simulink model "low_pass_filter"  (R2024b)
settings: Solver=FixedStepAuto  StartTime=0.0  StopTime=20  FixedStep=0.01  RelTol=1e-3
values from neighbouring files (symbols this model uses):
  alpha = 0.1    [lowpass_constants.m]
settings Model: Creator=AKhmad  LastModifiedBy=AKhmad

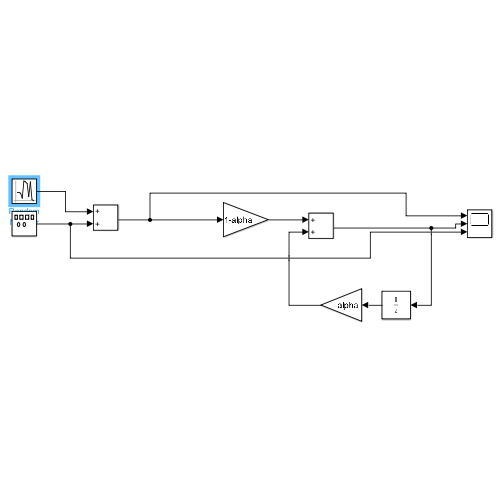
[thumbnail: Simulink's stored preview of the top-level diagram]
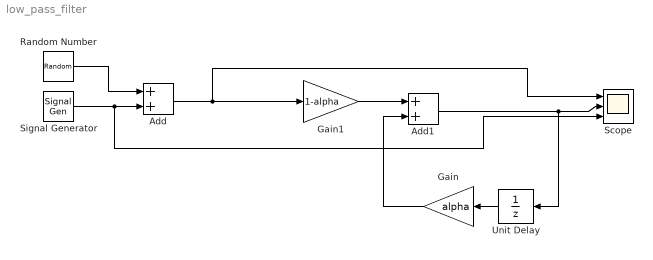
== system low_pass_filter ==
  Add : Sum
  Add1 : Sum
  Gain : Gain  Gain=alpha
  Gain1 : Gain  Gain=1-alpha
  Random Number : RandomNumber  SampleTime=0.1
  Scope : Scope  NumInputPorts=3
  Signal Generator : SignalGenerator  WaveForm=square  Amplitude=20  Frequency=0.1
  Unit Delay : UnitDelay  SampleTime=-1  HasFrameUpgradeWarning=on
  wires:
  Signal Generator/1 -> Scope/3, Add/2
  Random Number/1 -> Add/1
  Add/1 -> Scope/1, Gain1/1
  Unit Delay/1 -> Gain/1
  Gain/1 -> Add1/2
  Add1/1 -> Unit Delay/1, Scope/2
  Gain1/1 -> Add1/1
